simulink model "Missile_C_N"  (R2018b)
settings: Solver=ode4  StartTime=0.0  StopTime=5  FixedStep=Step_Size  RelTol=1e-3  EnableMultiTasking=on
InitFcn:
  | clc ;
  | clear all ;
  | close all ;
  | Missile_Data ;
  | Sim_Parameters ;
undefined symbols (not defined in the file): D, Tbl_ALPHAT, Tbl_CN_DEL_Y, Tbl_CN_PHIT, Tbl_CN_R, Tbl_MACH, XCG, XREF
libraries: simulink_extras x3
settings Model: Creator=e803534  LastModifiedBy=auten
settings OptimizationCC: LifeSpan=inf
settings DebuggingCC: UnconnectedInputMsg=none  UnconnectedOutputMsg=none  UnconnectedLineMsg=none  SFUnexpectedBacktrackingDiag=warning  SFNoUnconditionalDefaultTransitionDiag=warning
settings SFSimCC: SimUseLocalCustomCode=off
settings RTWCC: RTWUseLocalCustomCode=off
settings CodeAppCC: StateflowObjectComments=on
settings GRTTargetCC: TargetLangStandard=C89/C90 (ANSI)  GeneratePreprocessorConditionals=Disable all
settings ConfigComp: CovMetricSettings=dw  CovHtmlReporting=on  CovSaveCumulativeToWorkspaceVar=on  CovSaveSingleToWorkspaceVar=on  CovExternalEMLEnable=off

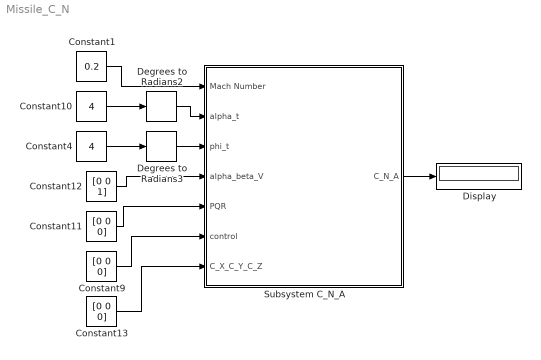
== system Missile_C_N ==
  Constant1 : Constant  Value=0.2
  Constant10 : Constant  Value=4
  Constant11 : Constant  Value=[0 0 0]
  Constant12 : Constant  Value=[0 0 1]
  Constant13 : Constant  Value=[0 0 0]
  Constant4 : Constant  Value=4
  Constant9 : Constant  Value=[0 0 0]
  Degrees to Radians2 : simulink_extras/Transformations/Degrees to Radians
  Degrees to Radians3 : simulink_extras/Transformations/Degrees to Radians
  Display : Display
  Subsystem C_N_A : Subsystem
  wires:
  Constant1/1 -> Subsystem C_N_A/1(Mach Number)
  Constant4/1 -> Degrees to Radians3/1
  Constant9/1 -> Subsystem C_N_A/6(control)
  Subsystem C_N_A/1(C_N_A) -> Display/1
  Constant10/1 -> Degrees to Radians2/1
  Constant11/1 -> Subsystem C_N_A/5(PQR)
  Constant12/1 -> Subsystem C_N_A/4(alpha_beta_V)
  Degrees to Radians2/1 -> Subsystem C_N_A/2(alpha_t)
  Degrees to Radians3/1 -> Subsystem C_N_A/3(phi_t)
  Constant13/1 -> Subsystem C_N_A/7(C_X_C_Y_C_Z)

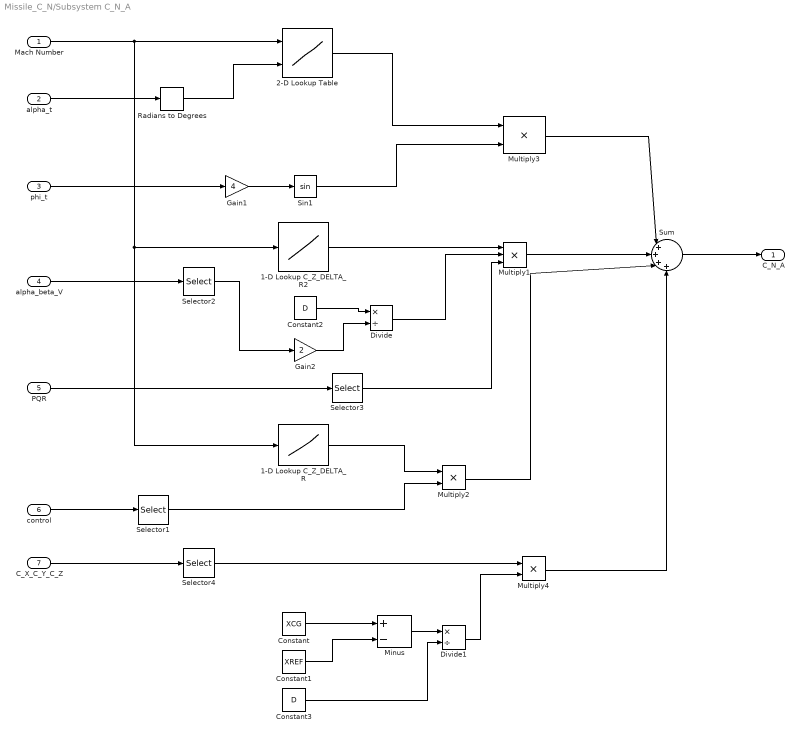
== system Missile_C_N/Subsystem C_N_A ==
  Mach Number : Inport
  alpha_t : Inport  Port=2
  phi_t : Inport  Port=3
  alpha_beta_V : Inport  Port=4
  PQR : Inport  Port=5
  control : Inport  Port=6
  C_X_C_Y_C_Z : Inport  Port=7
  1-D Lookup C_Z_DELTA_R : Lookup_n-D  NumberOfTableDimensions=1  BreakpointsForDimension1=Tbl_MACH  Table=Tbl_CN_DEL_Y  InternalRulePriority=Speed  RndMeth=Simplest  InputSameDT=on
  1-D Lookup C_Z_DELTA_R2 : Lookup_n-D  NumberOfTableDimensions=1  BreakpointsForDimension1=Tbl_MACH  Table=Tbl_CN_R  InternalRulePriority=Speed  RndMeth=Simplest  InputSameDT=on
  2-D Lookup Table : Lookup_n-D  BreakpointsForDimension1=Tbl_MACH  BreakpointsForDimension2=Tbl_ALPHAT  Table=Tbl_CN_PHIT  InternalRulePriority=Speed  RndMeth=Simplest  InputSameDT=on
  Constant : Constant  Value=XCG
  Constant1 : Constant  Value=XREF
  Constant2 : Constant  Value=D
  Constant3 : Constant  Value=D
  Divide : Product  Inputs=*/
  Divide1 : Product  Inputs=*/
  Gain1 : Gain  Gain=4
  Gain2 : Gain  Gain=2
  Minus : Sum  Inputs=+-
  Multiply1 : Product  Inputs=3
  Multiply2 : Product
  Multiply3 : Product
  Multiply4 : Product
  Radians to Degrees : simulink_extras/Transformations/Radians to Degrees
  Selector1 : Selector  InputPortWidth=3  IndexOptions=Index vector (dialog)  Indices=[3]  OutputSizes=1
  Selector2 : Selector  InputPortWidth=3  IndexOptions=Index vector (dialog)  Indices=[3]  OutputSizes=1
  Selector3 : Selector  InputPortWidth=3  IndexOptions=Index vector (dialog)  Indices=[3]  OutputSizes=1
  Selector4 : Selector  InputPortWidth=3  IndexOptions=Index vector (dialog)  Indices=[2]  OutputSizes=1
  Sin1 : Trigonometry
  Sum : Sum  Inputs=|++++
  C_N_A : Outport
  wires:
  2-D Lookup Table/1 -> Multiply3/1
  alpha_t/1 -> Radians to Degrees/1
  Sum/1 -> C_N_A/1
  Mach Number/1 -> 2-D Lookup Table/1, 1-D Lookup C_Z_DELTA_R/1, 1-D Lookup C_Z_DELTA_R2/1
  1-D Lookup C_Z_DELTA_R2/1 -> Multiply1/1
  1-D Lookup C_Z_DELTA_R/1 -> Multiply2/1
  Multiply2/1 -> Sum/3
  Sin1/1 -> Multiply3/2
  phi_t/1 -> Gain1/1
  Gain1/1 -> Sin1/1
  alpha_beta_V/1 -> Selector2/1
  Selector2/1 -> Gain2/1
  Divide/1 -> Multiply1/2
  PQR/1 -> Selector3/1
  Selector3/1 -> Multiply1/3
  control/1 -> Selector1/1
  Selector1/1 -> Multiply2/2
  C_X_C_Y_C_Z/1 -> Selector4/1
  Constant/1 -> Minus/1
  Constant1/1 -> Minus/2
  Constant2/1 -> Divide/1
  Minus/1 -> Divide1/1
  Constant3/1 -> Divide1/2
  Selector4/1 -> Multiply4/1
  Divide1/1 -> Multiply4/2
  Multiply4/1 -> Sum/4
  Multiply1/1 -> Sum/2
  Multiply3/1 -> Sum/1
  Radians to Degrees/1 -> 2-D Lookup Table/2
  Gain2/1 -> Divide/2
